simulink model "problem_3"  (R2019b)
settings: Solver=VariableStepAuto  StartTime=0.0  StopTime=20  RelTol=1e-3
settings Model: Creator=bhanu prasad  LastModifiedBy=bhanu prasad

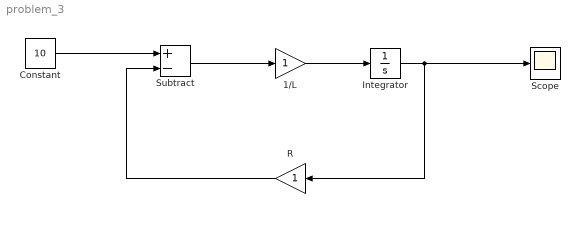
== system problem_3 ==
  1/L : Gain
  Constant : Constant  Value=10
  Integrator : Integrator
  R : Gain
  Scope : Scope
  Subtract : Sum  Inputs=+-
  wires:
  Constant/1 -> Subtract/1
  Subtract/1 -> 1/L/1
  1/L/1 -> Integrator/1
  Integrator/1 -> Scope/1, R/1
  R/1 -> Subtract/2
